simulink model "Phase2_Section3_integral_control"  (R2021b)
settings: Solver=VariableStepAuto  StartTime=0.0  StopTime=50  RelTol=1e-3
values from neighbouring files (symbols this model uses):
  A = [0 1 0; 244.86 -0.094 -26.29; 0 0 -250]    [Phase2_Section1.m]    (also in Phase2_Section2.m; Phase2_Section3.m; Phase2_Section4.m; Phase2_Section5.m)
  B = [0; 0; 5]    [Phase2_Section1.m]    (also in Phase2_Section2.m; Phase2_Section3.m; Phase2_Section4.m; Phase2_Section5.m)
  C = [1 0 0]    [Phase2_Section1.m]    (also in Phase2_Section2.m; Phase2_Section3.m; Phase2_Section4.m; Phase2_Section5.m)
  K = place(A_bar, B_bar, [-10, -20, -30,-40])    [Phase2_Section3.m]
settings Model: Creator=USER  LastModifiedBy=odeut

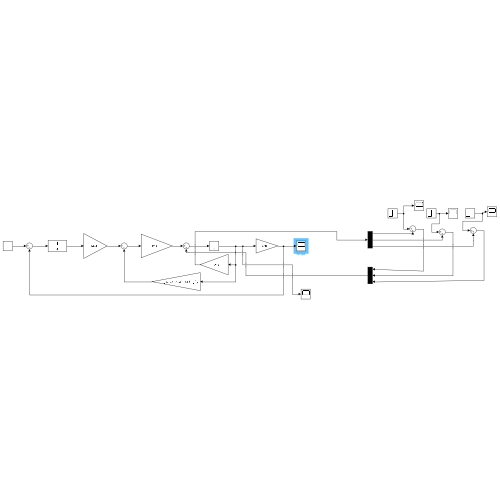
[thumbnail: Simulink's stored preview of the top-level diagram]
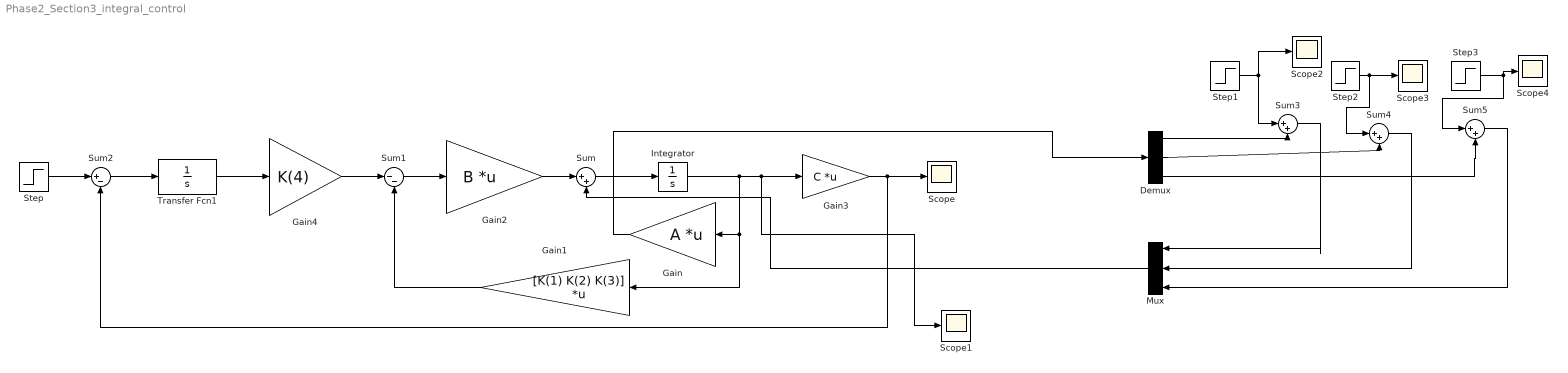
== system Phase2_Section3_integral_control ==
  Demux : Demux  Outputs=3
  Gain : Gain  Gain=A  Multiplication=Matrix(K*u)
  Gain1 : Gain  Gain=[K(1) K(2) K(3)]  Multiplication=Matrix(K*u)
  Gain2 : Gain  Gain=B  Multiplication=Matrix(K*u)
  Gain3 : Gain  Gain=C  Multiplication=Matrix(K*u)
  Gain4 : Gain  Gain=K(4)
  Integrator : Integrator
  Mux : Mux  Inputs=3
  Scope{,1..4} (5 alike) : Scope
  Step{,1..3} (4 alike) : Step  Time=0  SampleTime=0
  Sum{,3..5} (4 alike) : Sum  Inputs=|++
  Sum1 : Sum  Inputs=|--
  Sum2 : Sum  Inputs=|+-
  Transfer Fcn1 : TransferFcn  Denominator=[1 0]
  wires:
  Step/1 -> Sum2/1
  Sum2/1 -> Transfer Fcn1/1
  Gain4/1 -> Sum1/1
  Gain3/1 -> Sum2/2, Scope/1
  Gain2/1 -> Sum/1
  Transfer Fcn1/1 -> Gain4/1
  Sum1/1 -> Gain2/1
  Gain1/1 -> Sum1/2
  Sum/1 -> Integrator/1
  Integrator/1 -> Scope1/1, Gain3/1, Gain1/1, Gain/1
  Step1/1 -> Sum3/1, Scope2/1
  Sum3/1 -> Mux/1
  Demux/1 -> Sum3/2
  Demux/2 -> Sum4/2
  Step3/1 -> Sum5/1, Scope4/1
  Sum5/1 -> Mux/3
  Demux/3 -> Sum5/2
  Step2/1 -> Sum4/1, Scope3/1
  Sum4/1 -> Mux/2
  Gain/1 -> Demux/1
  Mux/1 -> Sum/2
